simulink model "chap6_7sim"  (Simulink 7.7)
settings: Solver=ode45  StartTime=0.0  StopTime=20  FixedStep=0.001  RelTol=1e-3
settings Model: Creator=hp  LastModifiedBy=ljk  ExtModeTrigMode=oneshot  ExtModeArmWhenConnect=off
settings DataIOCC: LimitDataPoints=off  SignalLoggingName=sigsOut
settings OptimizationCC: BooleanDataType=off  InitFltsAndDblsToZero=on
settings DebuggingCC: SaveWithParameterizedLinksMsg=none  SignalResolutionControl=TryResolveAllWithWarning  SolverPrmCheckMsg=none  MultiTaskDSMMsg=warning  MultiTaskCondExecSysMsg=none  StrictBusMsg=Warning
settings HardwareCC: TargetUnknown=on
settings RTWCC: IncludeERTFirstTime=on
settings GRTTargetCC: TargetFcnLib=ansi_tfl_tmw.mat

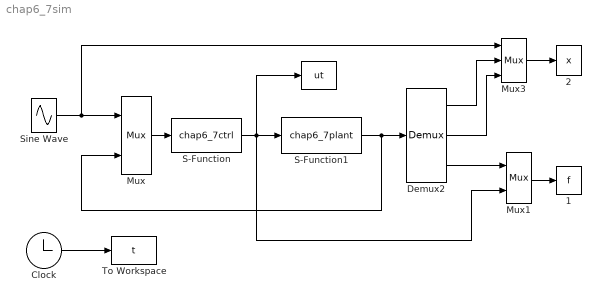
== system chap6_7sim ==
  " " : ToWorkspace  VariableName=ut  SampleTime=-1  SaveFormat=Array
  " 1" : ToWorkspace  VariableName=f  SampleTime=-1  SaveFormat=Array
  " 2" : ToWorkspace  VariableName=x  SampleTime=-1  SaveFormat=Array
  Clock : Clock
      settings: Decimation=10
  Demux2 : Demux  Outputs=3
  Mux : Mux  Inputs=2
  Mux1 : Mux  Inputs=2
  Mux3 : Mux  Inputs=3
  S-Function : S-Function  FunctionName=chap6_7ctrl  EnableBusSupport=off
  S-Function1 : S-Function  FunctionName=chap6_7plant  EnableBusSupport=off
  Sine Wave : Sin  SampleTime=0
  To Workspace : ToWorkspace  VariableName=t  SampleTime=-1  SaveFormat=Array
  wires:
  Mux/1 -> S-Function/1
  Mux3/1 -> " 2"/1
  S-Function/1 -> S-Function1/1, Mux1/2, " "/1
  Demux2/1 -> Mux3/2
  S-Function1/1 -> Demux2/1, Mux/2
  Clock/1 -> To Workspace/1
  Sine Wave/1 -> Mux3/1, Mux/1
  Mux1/1 -> " 1"/1
  Demux2/3 -> Mux1/1
  Demux2/2 -> Mux3/3
